simulink model "learning_conrtol"  (R2021a)
settings: Solver=VariableStepAuto  StartTime=0.0  StopTime=10.0  RelTol=1e-3
settings Model: Creator=061  LastModifiedBy=061

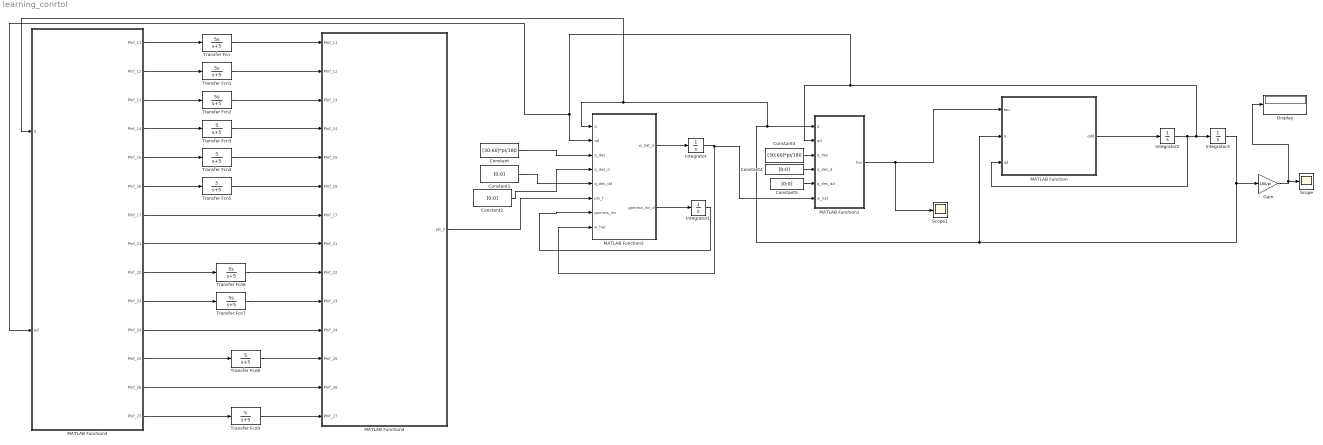
== system learning_conrtol ==
  Constant : Constant  Value=[30;60]*pi/180
  Constant{1..2,4..5} (4 alike) : Constant  Value=[0;0]
  Constant3 : Constant  Value=[30;60]*pi/180
  Display : Display
  Gain : Gain  Gain=180/pi
  Integrator : Integrator  InitialCondition=rand(7,1)
  Integrator1 : Integrator  InitialCondition=3*eye(7,7)
  Integrator2 : Integrator  InitialCondition=zeros(2,1)
  Integrator3 : Integrator  InitialCondition=zeros(2,1)
  MATLAB Function : MATLAB Function  TreatAsAtomicUnit=on
  MATLAB Function1 : MATLAB Function  TreatAsAtomicUnit=on
  MATLAB Function2 : MATLAB Function  TreatAsAtomicUnit=on
  MATLAB Function3 : MATLAB Function  TreatAsAtomicUnit=on
  MATLAB Function4 : MATLAB Function  TreatAsAtomicUnit=on
  Scope : Scope
  Scope1 : Scope
  Transfer Fcn{,1..2,6..7} (5 alike) : TransferFcn  Numerator=[5 0]  Denominator=[1 5]
  Transfer Fcn{3..5,8..9} (5 alike) : TransferFcn  Numerator=[5]  Denominator=[1 5]
  wires:
  MATLAB Function3/1(Phif_11) -> Transfer Fcn/1
  MATLAB Function3/2(Phif_12) -> Transfer Fcn1/1
  MATLAB Function3/3(Phif_13) -> Transfer Fcn2/1
  MATLAB Function3/4(Phif_14) -> Transfer Fcn3/1
  MATLAB Function3/5(Phif_15) -> Transfer Fcn4/1
  MATLAB Function3/6(Phif_16) -> Transfer Fcn5/1
  MATLAB Function3/9(Phif_22) -> Transfer Fcn6/1
  MATLAB Function3/10(Phif_23) -> Transfer Fcn7/1
  MATLAB Function3/12(Phif_25) -> Transfer Fcn8/1
  MATLAB Function3/14(Phif_27) -> Transfer Fcn9/1
  Transfer Fcn/1 -> MATLAB Function4/1(Phif_11)
  Transfer Fcn1/1 -> MATLAB Function4/2(Phif_12)
  Transfer Fcn2/1 -> MATLAB Function4/3(Phif_13)
  Transfer Fcn3/1 -> MATLAB Function4/4(Phif_14)
  Transfer Fcn4/1 -> MATLAB Function4/5(Phif_15)
  Transfer Fcn5/1 -> MATLAB Function4/6(Phif_16)
  MATLAB Function3/7(Phif_17) -> MATLAB Function4/7(Phif_17)
  MATLAB Function3/8(Phif_21) -> MATLAB Function4/8(Phif_21)
  Transfer Fcn6/1 -> MATLAB Function4/9(Phif_22)
  Transfer Fcn7/1 -> MATLAB Function4/10(Phif_23)
  MATLAB Function3/11(Phif_24) -> MATLAB Function4/11(Phif_24)
  Transfer Fcn8/1 -> MATLAB Function4/12(Phif_25)
  MATLAB Function3/13(Phif_26) -> MATLAB Function4/13(Phif_26)
  Transfer Fcn9/1 -> MATLAB Function4/14(Phif_27)
  MATLAB Function4/1(phi_F) -> MATLAB Function2/6(phi_f)
  MATLAB Function2/1(w_hat_d) -> Integrator/1
  MATLAB Function2/2(gamma_inv_d) -> Integrator1/1
  Integrator1/1 -> MATLAB Function2/7(gamma_inv)
  MATLAB Function1/1(tau) -> Scope1/1, MATLAB Function/1(tau)
  MATLAB Function/1(qdd) -> Integrator2/1
  Integrator3/1 -> MATLAB Function/2(q), MATLAB Function3/1(q), MATLAB Function2/1(q), MATLAB Function1/1(q), Gain/1
  Integrator/1 -> MATLAB Function2/8(w_hat), MATLAB Function1/6(w_hat)
  Integrator2/1 -> MATLAB Function/3(qd), MATLAB Function3/2(qd), MATLAB Function2/2(qd), MATLAB Function1/2(qd), Integrator3/1
  Constant/1 -> MATLAB Function2/3(q_des)
  Constant2/1 -> MATLAB Function2/4(q_des_d)
  Constant3/1 -> MATLAB Function1/3(q_des)
  Constant4/1 -> MATLAB Function1/4(q_des_d)
  Constant5/1 -> MATLAB Function1/5(q_des_dd)
  Gain/1 -> Display/1, Scope/1
  Constant1/1 -> MATLAB Function2/5(q_des_dd)

== matlab function learning_conrtol/MATLAB Function1 ==
  data: q input; tau output; qd input; q_des input; q_des_d input; q_des_dd input; w_hat input
function tau = fcn(q,qd,q_des,q_des_d,q_des_dd,w_hat)
g=9.81;
alph=5;
lambda=2*eye(2);
kc=10*eye(2);
e=q_des-q;
ed=q_des_d-qd;
ef=ed+lambda*e;
v=q_des_d+lambda*e;
vd=q_des_dd+lambda*ed;
phi=[vd(1) vd(2) (2*vd(1)+vd(2))*cos(q(2))-(qd(2)*v(1)+(qd(1)+qd(2))*v(2))*sin(q(2)) g*cos(q(1)) g*cos(q(1)+q(2)) qd(1) 0;
    0 vd(1)+vd(2) vd(1)*cos(q(2))+qd(1)*v(1)*sin(q(2)) 0 g*cos(q(1)+q(2)) 0 qd(2)]';
tau=kc*ef+phi'*w_hat

== matlab function learning_conrtol/MATLAB Function ==
  data: tau input; qdd output; q input; qd input
function qdd = fcn(tau,q,qd)

q1=q(1);
q2=q(2);

q1d=qd(1);
q2d=qd(2);




m1=2;
m2=1.4;

I1=.5;
I2=.1;

l1=.8;
l2=.8;

lc1=.4;
lc2=.4;


g=9.81;

kv1=.8;
kv2=1.6;
D=[kv1 0;0 kv2];




d11=m1*lc1^2+I1+I2+m2*(l1^2+lc2^2+2*l1*lc2*cos(q2));
d12=m2*lc2^2+I2+m2*l2*lc2*cos(q2);
d21=m2*lc2^2+I2+m2*l2*lc2*cos(q2);
d22=m2*lc2^2+I2;

c11=-m2*l1*lc2*sin(q2)*q2d;
c12=-m2*l1*lc2*sin(q2)*(q1d+q2d);
c21=m2*l1*lc2*sin(q2)*q1d;
c22=0;

g11=m1*lc1*g*cos(q1)+m2*g*(lc2*cos(q1+q2)+l1*cos(q1));
g21=m2*lc2*g*cos(q1+q2);

M=[d11,d12;d21,d22];
C=[c11 c12;c21 c22];
G=[g11;g21];
qdd=pinv(M)*(tau-C*qd-D*qd-G);

== matlab function learning_conrtol/MATLAB Function2 ==
  data: q input; w_hat_d output; qd input; q_des input; q_des_d input; q_des_dd input; phi_f input; gamma_inv input; w_hat input; gamma_inv_d output
function [w_hat_d,gamma_inv_d] = fcn(q,qd,q_des,q_des_d,q_des_dd,phi_f,gamma_inv,w_hat)

m1=2;
m2=1.4;

I1=.5;
I2=.1;

l1=.8;
l2=.8;

lc1=.4;
lc2=.4;


g=9.81;

kv1=.8;
kv2=1.6;
w1=I1+m1*lc1^2+m2*l1^2+m2*lc2^2;
w2=m2*lc2^2+I2;
w3=m2*l1*lc2;
w4=m1*lc1+m2*l1;
w5=m2*lc2;
w6=kv1;
w7=kv2;
w=[w1,w2,w3,w4,w5,w6,w7]';
landa_0=1
k_0=3
kappa=1;
g=9.81;
alph=5;
lambda=2*eye(2);
kc=10*eye(2);
e=q_des-q;
ed=q_des_d-qd;
ef=ed+lambda*e;
v=q_des_d+lambda*e;
vd=q_des_dd+lambda*ed;

phi=[vd(1) vd(2) (2*vd(1)+vd(2))*cos(q(2))-(qd(2)*v(1)+(qd(1)+qd(2))*v(2))*sin(q(2)) g*cos(q(1)) g*cos(q(1)+q(2)) qd(1) 0;
    0 vd(1)+vd(2) vd(1)*cos(q(2))+qd(1)*v(1)*sin(q(2)) 0 g*cos(q(1)+q(2)) 0 qd(2)]';

gamma=pinv(gamma_inv);

landa=landa_0*(1-(norm(gamma,2)/k_0));

gamma_inv_d=(-landa*gamma_inv)+(phi_f*(phi_f)');

epsilon=(phi_f)'*w-(phi_f)'*w_hat;

w_hat_d=gamma*(phi*ef+kappa*phi_f*epsilon);

== matlab function learning_conrtol/MATLAB Function3 ==
  data: q input; Phif_11 output; qd input; Phif_12 output; Phif_13 output; Phif_14 output; Phif_15 output; Phif_16 output; Phif_17 output; Phif_21 output; Phif_22 output; Phif_23 output; Phif_24 output; Phif_25 output; Phif_26 output; Phif_27 output
function  [Phif_11,Phif_12,Phif_13,Phif_14,Phif_15,Phif_16,Phif_17,Phif_21,Phif_22,Phif_23,Phif_24,Phif_25,Phif_26,Phif_27]= fcn(q,qd)
g=9.81
Phif_11=qd(1);
Phif_12=qd(2);
Phif_13=(2*qd(1)+qd(2))*cos(q(2));
Phif_14=g*cos(q(1));
Phif_15=g*cos(q(1)+q(2));
Phif_16=qd(1);
Phif_17=0;
Phif_21=0;
Phif_22=qd(1)+qd(2);
Phif_23=qd(1)*cos(q(2))+qd(1)*sin(q(2))*(qd(1)+qd(2));
Phif_24=0;
Phif_25=g*cos(q(1)+q(2));
Phif_26=0;
Phif_27=qd(2);

== matlab function learning_conrtol/MATLAB Function4 ==
  data: Phif_11 input; phi_F output; Phif_12 input; Phif_13 input; Phif_14 input; Phif_15 input; Phif_16 input; Phif_17 input; Phif_21 input; Phif_22 input; Phif_23 input; Phif_24 input; Phif_25 input; Phif_26 input; Phif_27 input
function phi_F = fcn(Phif_11,Phif_12,Phif_13,Phif_14,Phif_15,Phif_16,Phif_17,Phif_21,Phif_22,Phif_23,Phif_24,Phif_25,Phif_26,Phif_27)
phi_F=[Phif_11,Phif_12,Phif_13,Phif_14,Phif_15,Phif_16,Phif_17;Phif_21,Phif_22,Phif_23,Phif_24,Phif_25,Phif_26,Phif_27]';
